simulink model "bmw_i3_model"  (R2025b)
settings: Solver=ode4  StartTime=0.0  StopTime=1179  FixedStep=1  RelTol=1e-3
settings Model: Creator=Piyush  LastModifiedBy=Piyush

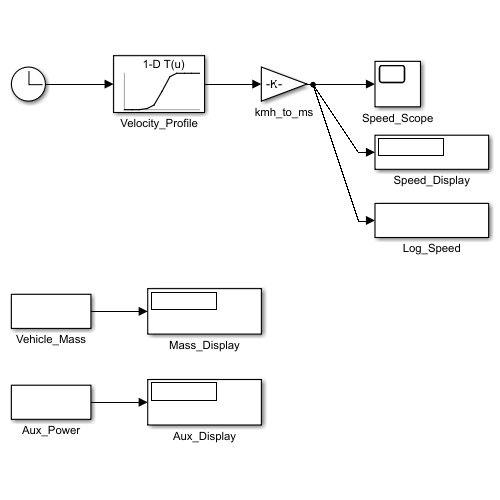
[thumbnail: Simulink's stored preview of the top-level diagram]
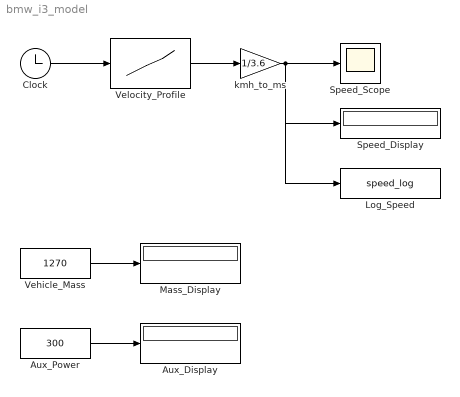
== system bmw_i3_model ==
  Aux_Display : Display
  Aux_Power : Constant  Value=300
  Clock : Clock
  Log_Speed : ToWorkspace  VariableName=speed_log  SampleTime=-1
  Mass_Display : Display
  Speed_Display : Display
  Speed_Scope : Scope
  Vehicle_Mass : Constant  Value=1270
  Velocity_Profile : Lookup_n-D  NumberOfTableDimensions=1  BreakpointsForDimension1=[-5:5]  Table=tanh([-5:5])  InternalRulePriority=Speed  RndMeth=Simplest
  kmh_to_ms : Gain  Gain=1/3.6
  wires:
  Clock/1 -> Velocity_Profile/1
  Velocity_Profile/1 -> kmh_to_ms/1
  kmh_to_ms/1 -> Speed_Scope/1, Speed_Display/1, Log_Speed/1
  Vehicle_Mass/1 -> Mass_Display/1
  Aux_Power/1 -> Aux_Display/1
